simulink model "CONTROL_POSICION_Robotica"  (Simulink 7.7)
settings: Solver=ode45  StartTime=0.0  StopTime=inf  RelTol=1e-3
settings Model: Creator=JohnConstantine  LastModifiedBy=JohnConstantine

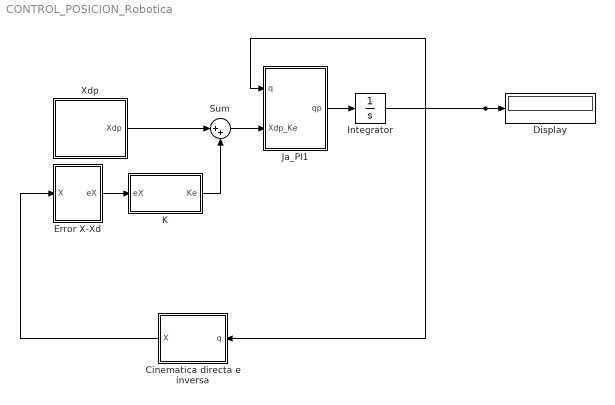
== system CONTROL_POSICION_Robotica ==
  Cinematica directa e inversa : Stateflow chart  TreatAsAtomicUnit=on
  Display : Display
  Error X-Xd : Stateflow chart  TreatAsAtomicUnit=on
  Integrator : Integrator  InitialCondition=45
  Ja_PI1 : Stateflow chart  TreatAsAtomicUnit=on
  K : Stateflow chart  TreatAsAtomicUnit=on
  Sum : Sum  Inputs=|++
  Xdp : Stateflow chart  TreatAsAtomicUnit=on
  wires:
  Integrator/1 -> Cinematica directa e inversa/1(q), Ja_PI1/1(q), Display/1
  Cinematica directa e inversa/1(X) -> Error X-Xd/1(X)
  Xdp/1(Xdp) -> Sum/1
  Error X-Xd/1(eX) -> K/1(eX)
  K/1(Ke) -> Sum/2
  Sum/1 -> Ja_PI1/2(Xdp_Ke)
  Ja_PI1/1(qp) -> Integrator/1

== matlab function Error X-Xd ==
  data: X input double; eX output double
function eX  = Control(X)  %donde X es igual a los valores de X=[p ; Theta] ; un vector de 6 valores transpuestos


%%%% Pose deseada y sus derivadas %%%%%%%% 
Xd=[0 0 0 0 0 0].';
Xpd=[0 0 0 0 0 0].';
%%% Errores de posición y velocidad %%%
eX=X-Xd;
exp=Xp-Xpd;

== matlab function K ==
  data: eX input double; Ke output double

function Ke  = Control(eX)


kp=100*eye(6);
kd=10*eye(6); 

Ke=-kp*eX; %-kd*Ja*qp;

== matlab function Cinematica directa e inversa ==
  data: q input double; X output double
function X  =mgdFalange(q)

q1=q(1);%q1=d1
q2=q(2);
q3=q(3);
q4=q(4);

d2=12.0349;
a2=7.907;
a3=8.862;
a4=15;
a5=8.862;
a6=15;

 MGD=[ -cos(q3 + q4)*sin(q2),  sin(q3 + q4)*sin(q2), cos(q2),                                         -sin(q2)*(a2 + a5*cos(q3 + q4) + a6*cos(q3 + q4) + a3*cos(q3) + a4*cos(q3));...
               -sin(q3 + q4),         -cos(q3 + q4),       0,                                                  - d2 - a5*sin(q3 + q4) - a6*sin(q3 + q4) - a3*sin(q3) - a4*sin(q3);...
        cos(q3 + q4)*cos(q2), -sin(q3 + q4)*cos(q2), sin(q2), q1 + a2*cos(q2) + cos(q2)*cos(q3)*(a3 + a4) - cos(q2)*sin(q3)*sin(q4)*(a5 + a6) + cos(q2)*cos(q3)*cos(q4)*(a5 + a6);...
                           0,                     0,       0,                                                                                                                  1];
                                                                                                                                                                                                                                                                                 
H=MGD;

Pxyz=[MGD(1,4) MGD(2,4) MGD(3,4)].';

% r21=H(2,1);
% r11=H(1,1);
% r31=H(3,1);
% r32=H(3,2);
% r33=H(3,3);
%rt=[H(2,1) H(1,1) H(3,1) H(3,2) H(3,3);];%Las posiciones de la matriz de rotacion de los angulos de EULER y RPY para el calculo de alpha, gamma, theta

al=atan2(r21,r11);
ga=atan2(-r31,sqrt(r32^2+r33^2));
th=atan2(r32,r33);

Theta=[al ga th].'; % valores de theta
X=[Pxyz; 
   Theta]

== matlab function Xdp ==
  data: Xdp output double
function Xdp  = Xdp  %donde X es igual a los valores de X=[p ; Theta] ; un vector de 6 valores transpuestos


%%%% Pose deseada y sus derivadas %%%%%%%% 
Xdp= [  cos(t)*.5   1/20   -sin(t)*.5   0   0   0].';

== matlab function Ja_PI1 ==
  data: q input double; qp output double; Xdp_Ke input double

function qp= Control(q,Xdp_Ke)
q1=q(1);%q1=d1
q2=q(2);
q3=q(3);
q4=q(4);

qt=[q1; q2; q3; q4].';
% q1p=qp(1);
% q2p=qp(2);
% q3p=qp(3);
% q4p=qp(4);

d2=12.0349;
a2=7.907;
a3=8.862;
a4=15;
a5=8.862;
a6=15;

%%%%%%%%%%%%%%%%%%%%%%%%%%%%%%%%%%%%%%%%%%
%%CALCULO DEL MODELO GEOMETRICO DIRECTO %%
%%%%%%%%%%%%%%%%%%%%%%%%%%%%%%%%%%%%%%%%%%
%% q1=d1;

%DHmatrix(th,d,a,al)
 A1=DHmatrix(0,q1,0,pi/2);
 A2=DHmatrix(q2+pi/2,d2,a2,pi/2);
 A3=DHmatrix(q3,0,a3+a4,0);
 A4=DHmatrix(q4,0,a5+a6,0);

 T1=A1;
 T12=A1*A2;
 T13=A1*A2*A3;
 T14=A1*A2*A3*A4;

H=simple(T14);

 
%%%%%%%%%%%%%%%%%%%%%%%%%%%%%%%%%%%%%%%%%%%%%%%%%%%%%%%%%%
%%                 CALCULO DE JACOBIANOS                %%
%%%%%%%%%%%%%%%%%%%%%%%%%%%%%%%%%%%%%%%%%%%%%%%%%%%%%%%%%%
%A PARTIR DE LA VELOCIDAD ANGULAR DEL JACOBIANO GEOMETRICO 
%DONDE Jg=[I     0 ]*Ja       Ja=Jacobiano Analitico Jg=Jacobiano geometrico 
%         [0 T(phi)]          T(phi)=Son los vectores (columna 1, 2 , 3) de cada multiplicación de transformacion de
%                             las configuraciones que uno elija de la rotacion xyz, zyz, etc.

%POR LO TANTO Ja=[I      0     ]*Jg
%                [0 inv(T(phi))]

%% CALCULO DE LOS ANGULOS DE EULER A PARTIR DE LA MATRIZ DE TRANSFORMACIÓN HOMOGENEA (solo tomo la matriz de rotacion 3x3), Y UTILIZANDO LA MATRIZ XYZ DE LOS ANGULOS DE EULER
%% LOS VALORES OBTENIDOS DE al, ga, th SE SUSTITUYEN EN TIEMPO REAL EN LA MATRIZ DE Tphi PARA OBTENER LOS VALORES DE T(phi)
 r21=H(2,1);
 r11=H(1,1);
 r31=H(3,1);
 r32=H(3,2);
 r33=H(3,3);

  al=atan2(r21,r11);
  ga=atan2(-r31,sqrt(r32^2+r33^2));
  th=atan2(r32,r33);


%%%%%%%%%%%%%%%%%%%%%%%%%%%%%%%%%%%%%%%%%%%%%
%% MATRIZ T(phi) PARA LA CONFIGURACION RPY %%
%%%%%%%%%%%%%%%%%%%%%%%%%%%%%%%%%%%%%%%%%%%%%

%PARA VER EL CODIGO DE COMO SE OBTIENE XYZ IR AL PROGRAMA
%MATRIZ_RPY

%% Matriz B o T(phi) obtenida a partir de los angulos de Euler (XYZ) de la rotacion RPY
Tphi = [ 0, -sin(th), cos(ga)*cos(th);
         0,  cos(th), cos(ga)*sin(th);
         1,        0,       -sin(ga)]


%% Valores obtenidos del programa JACOBIANO GEOMETRICO

 Jg=[0, -cos(q2)*(a2 + a5*cos(q3 + q4) + a6*cos(q3 + q4) + a3*cos(q3) + a4*cos(q3)),  sin(q2)*(a5*sin(q3 + q4) + a6*sin(q3 + q4) + a3*sin(q3) + a4*sin(q3)),  sin(q3 + q4)*sin(q2)*(a5 + a6);
    0,                                                                           0,          - a5*cos(q3 + q4) - a6*cos(q3 + q4) - a3*cos(q3) - a4*cos(q3),         -cos(q3 + q4)*(a5 + a6);
    1, -sin(q2)*(a2 + a5*cos(q3 + q4) + a6*cos(q3 + q4) + a3*cos(q3) + a4*cos(q3)), -cos(q2)*(a5*sin(q3 + q4) + a6*sin(q3 + q4) + a3*sin(q3) + a4*sin(q3)), -sin(q3 + q4)*cos(q2)*(a5 + a6);
    0,                                                                           0,                                                                cos(q2),                         cos(q2);
    0,                                                                          -1,                                                                      0,                               0;
    0,                                                                           0,                                                                sin(q2),                         sin(q2)]


%%%%%%%%%%%%%%%%%%%%%%%%%%%%%%%%%%%%%%%%%%%%%%%%%%%%%%%%%%%%%%%%%%%%%%%%%%%%%%%%%%%%%%
%% OBTENCIÓN DE LA MATRIZ DEL JACOBIANO ANALITICO A PARTIR DEL JACOBIANO GEOMETRICO %%
%%%%%%%%%%%%%%%%%%%%%%%%%%%%%%%%%%%%%%%%%%%%%%%%%%%%%%%%%%%%%%%%%%%%%%%%%%%%%%%%%%%%%%
%  Ja=[I      0     ]*Jg
%     [0 inv(T(phi))]

iTphi=inv(Tphi);

Ta_phi=[ eye(3)    zeros(3,3); %[I     0    ]
        zeros(3,3)   iTphi]   %[0 inv(Tphi)]

Ja=simple(Ta_phi*Jg) %ES UNA MATRIZ DE TAMAÑO 6x4

%%%%%%%%%%%%%%%%%%%%%%%%%%%%%%%%%%%%%%%%%%%%%%%%%%%%%%%%%%%%%%%%%%%%
%% JACOBIANA INVERSA POR EL METODO DE LA PSEUDO-INVERSA IZQUIERDA %%
%% DONDE m>n ES DECIR TIENE MAS FILA(6) QUE COLUMNAS(4)           %% 
%%%%%%%%%%%%%%%%%%%%%%%%%%%%%%%%%%%%%%%%%%%%%%%%%%%%%%%%%%%%%%%%%%%%

 J_PI=(Ja.'*Ja + lambda*eye(4))\Ja.';
 
 qp=J_PI*qt*(Xdp_Ke);
